simulink model "youhua_1226"  (R2017b)
settings: Solver=ode1  StartTime=0.0  StopTime=Inf  FixedStep=0.0002  RelTol=1e-3
PreLoadFcn:
  | initFun_4P.m
PostLoadFcn:
  | , if any(exist('dsrtsu_mdlpostloadfcn', 'file') == [2, 3, 6]), try dsrtsu_mdlpostloadfcn('Execute', bdroot); catch fprintf('Error in PostLoadFcn (dsrtsu_mdlpostloadfcn) for model "%s":\n %s\n', bdroot, lasterr); end, end,
InitFcn:
  | initFun_4P
undefined symbols (not defined in the file): CMAES_B_initial, CMAES_C_initial, CMAES_chiN_initial, CMAES_counteval_initial, CMAES_D_initial, CMAES_eigeneval_initial, CMAES_invsqrtC_initial, CMAES_pc_initial, CMAES_ps_initial, CMAES_sigma_initial, CMAES_xmean_initial
libraries: rti1202lib_adc_class1 x20, simulink x8, dsparch4 x6, rti1202serlib x4, rti1202lib_dio_class1 x4, dsextras x3, rtiemclib x2, rti1202lib_dac_class1 x1, rtitasklib x1
(part 5 of 6)

== matlab function youhua_1226/CONTROL/Control and Display/State Transition ==
  data: state_output output; stride_T output; buttons input; digital_inputs input; state_input input; analog_inputs input; user_inputs input; state_variables input; current_time input; ABL_user_inputs input; max_ankle_pos input; current_state_time output
function [state_output, stride_T, current_state_time] = fcn(buttons, digital_inputs, state_input,...
    analog_inputs, user_inputs, state_variables, current_time, ...
    ABL_user_inputs, max_ankle_pos)



%State definitions
idle_state	=	0;
calibration_state	=   1;
stance_state   =   2;
swing_state     =   3;
step_state  =   4;
slack_state = 5;
pos_track_state = 6;
%#eml

tracksize = 5;




foot_switch     =   digital_inputs(1);


bt_set_zero     =   buttons(1);
bt_walk         =   buttons(2);
bt_stop         =   buttons(3);
bt_step         =   buttons(4);
bt_slack        =   buttons(5);
bt_pos_test     =   buttons(6);

% measured_force = analog_inputs(4);
measured_force = state_variables(7);
ankle_pos = state_variables(3);
measured_torque = state_variables(6);

slack_force = user_inputs(5);
slack_length = user_inputs(22);
planter_low_limit = user_inputs(77);
walk_control_mode = user_inputs(21);

%当前状态持续时间
current_state_time = state_variables(21)-state_variables(23);

current_state = state_input(1);
stop_pos_prev = state_input(2);
slack_pos_prev = state_input(3);
stance_end_pos_prev = state_input(4);
stance_period_prev = state_input(5);
flag_dorsi_plantar_prev = state_input(6);
temp_ankle_pos1_prev = state_input(7);
temp_ankle_pos2_prev = state_input(8);
temp_ankle_pos3_prev = state_input(9);
temp_ankle_pos4_prev = state_input(10);
temp_ankle_pos5_prev = state_input(11);
stance_index_prev = state_input(12);
stride_time_prev = state_input(13);
step_start_time_prev = state_input(14);
dorsi_end_pos_prev = state_input(15);
ABL_ankle_index_prev = state_input(16);




state_output = state_input;
stop_pos = stop_pos_prev;
slack_pos = slack_pos_prev;
stance_end_pos = stance_end_pos_prev;
stance_period = stance_period_prev;
flag_dorsi_plantar = flag_dorsi_plantar_prev;
temp_ankle_pos1 = temp_ankle_pos2_prev;
temp_ankle_pos2 = temp_ankle_pos3_prev;
temp_ankle_pos3 = temp_ankle_pos4_prev;
temp_ankle_pos4 = temp_ankle_pos5_prev;
temp_ankle_pos5 = state_variables(3);
stance_index = stance_index_prev;
stride_time = stride_time_prev;
%---------------------
stride_T = stride_time;
%---------------------------
ABL_ankle_index = ABL_ankle_index_prev;

if(stride_time <0.7)
    stride_time = 0.7;
elseif(stride_time>1.5)
    stride_time =1.5;
end
step_start_time = step_start_time_prev;
dorsi_end_pos = dorsi_end_pos_prev;

ABL_ankle_min = ABL_user_inputs(1);
ABL_ankle_res = ABL_user_inputs(2);
ABL_or_TBL = ABL_user_inputs(3);


% ABL_ankle_index = stance_index_prev;
ABL_ankle_index = floor((ankle_pos-ABL_ankle_min)/ABL_ankle_res)+1;


switch current_state
    case idle_state
        if bt_set_zero  ==  1
            next_state = calibration_state;
        elseif bt_slack  == 1
            next_state = slack_state;
            slack_pos = state_variables(4);
        elseif bt_walk	==  1
            next_state = swing_state;
        elseif bt_step  ==  1
            next_state = step_state;
        elseif bt_pos_test ==1
            next_state = pos_track_state;
        else
            next_state = idle_state;
            %             stop_pos = state_variables(4);
        end
    case calibration_state
        if bt_stop == 1
            next_state = idle_state;
            stop_pos = state_variables(4);
        elseif measured_torque < slack_force % less than 2 lbs
            next_state = calibration_state;
        else
            next_state = idle_state;
            stop_pos = state_variables(4);
        end
    case stance_state
        %---------------

        %---------------
        if bt_stop	==	1
            next_state = idle_state;
            stop_pos = state_variables(4);
            flag_dorsi_plantar = 0;
        elseif bt_slack  == 1
            next_state = slack_state;
            slack_pos = state_variables(4);
            flag_dorsi_plantar = 0;
            %         elseif (current_state_time >=0.6*stride_time && temp_ankle_pos5<temp_ankle_pos4 && temp_ankle_pos5<temp_ankle_pos4 && measured_force<planter_low_limit)
%         elseif (current_state_time >=0.65*stride_time ||
%         ankle_pos>max_ankle_pos) $$$$$$$$$$
            elseif (current_state_time >=0.65*stride_time)
            next_state = swing_state;
            stance_end_pos = state_variables(4);
            stance_period = current_state_time;
            flag_dorsi_plantar = 0;
        elseif current_state_time<0.30*stride_time
            next_state = stance_state;
            stance_index = stance_index +1;
            flag_dorsi_plantar = 0;
        else
            stance_index = stance_index+1;
            next_state = stance_state;
            if flag_dorsi_plantar == 0
                if(temp_ankle_pos4>temp_ankle_pos3 && temp_ankle_pos5>temp_ankle_pos4)
                    flag_dorsi_plantar = 1;
                    dorsi_end_pos = state_variables(3);
                end
            end
        end
    case swing_state
        %---------

        %---------------
        
        if bt_stop == 1
            next_state = idle_state;
            stop_pos = state_variables(4);
        elseif bt_slack  == 1
            next_state = slack_state;
            slack_pos = state_variables(4);
        elseif foot_switch ==   1
            if current_state_time>0.15*stride_time
%                 if current_state_time>0.15

                next_state = stance_state;
                stance_index = 1;
                stride_time = (current_time - step_start_time+stride_time+stride_time_prev)/3;
                step_start_time = current_time;
            else
                next_state = swing_state;
            end
        else
            next_state = swing_state;
        end
    case step_state
        if bt_stop == 1
            next_state = idle_state;
            stop_pos = state_variables(4);
        elseif bt_slack  == 1
            next_state = slack_state;
            slack_pos = state_variables(4);
        else
            next_state = step_state;
        end
    case slack_state
        if bt_stop == 1
            next_state = idle_state;
            stop_pos = state_variables(4);
        elseif (abs(state_variables(4)-slack_pos-slack_length)<1)
            next_state = idle_state;
            stop_pos = state_variables(4);
        else
            next_state = slack_state;
        end
    case pos_track_state
        if bt_stop == 1
            next_state = idle_state;
            stop_pos = state_variables(4);
        elseif bt_slack  == 1
            next_state = slack_state;
            slack_pos = state_variables(4);
        else
            next_state = pos_track_state;
        end
    otherwise
        next_state  = current_state;
end

state_output(1) = next_state;
state_output(2) = stop_pos;
state_output(3) = slack_pos;
state_output(4) = stance_end_pos;
state_output(5) = stance_period;
state_output(6) = flag_dorsi_plantar;
state_output(7) = temp_ankle_pos1;
state_output(8) = temp_ankle_pos2;
state_output(9) = temp_ankle_pos3;
state_output(10) = temp_ankle_pos4;
state_output(11) = temp_ankle_pos5;

%     case 0
%         if flag_dorsi_planter==0
%         state_output(12) = ABL_ankle_index;
%         else
%             state_output(12) = ABL_ankle_index + 300;
%         end;
%     case 1
%     state_output(12) = stance_index;
%     otherwise
state_output(12) = stance_index;
state_output(13) = stride_time;
state_output(14) = step_start_time;
state_output(15) = dorsi_end_pos;
if flag_dorsi_plantar==0
    state_output(16) = ABL_ankle_index;
else
    state_output(16) = ABL_ankle_index + 300;
end
return

== matlab function youhua_1226/CONTROL/Control and Display/OutputBlock/Display and Recording ==
  data: current_state input; state output; state_variables input; motor_velocity input; desired_velocity output; zero_ankle_pos output; zero_motor_pos output; ankle_pos output; motor_pos output; desired_torque output; measured_torque output; load_force output; load_angle output; load_pivot_distance output; delta_motor_pos output; slack_motor_pos output; torque_error output; Kp output; ankle_vel output; motor_vel output; motor_acc output; Kd output; Ki output; controller_type output; Kc output; current_time output; state_start_time output; curve_id output; Kpp output; accumulated_torque_error output; desired_motor_pos output; walk_control_mode output; prev_step_accumulated_error output; curr_step_accumulated_error output; learning_control_input output; learning_control_input2 output; Kp2 output; Kl output; Kl2 output; flag_d_p output; gamma output; Lce output; Lmtu output; FL output; Fpe output; ACT output; STIM output; Fmtu output; Lcedot output; learned_value output; learned_avg output; accumulated_pos_error output; gamma1 output; gamma2 output; gamma3 output; gamma4 output
function [state, desired_velocity, zero_ankle_pos,  zero_motor_pos,...
    ankle_pos,motor_pos,desired_torque,measured_torque,load_force,...
    load_angle, load_pivot_distance,delta_motor_pos,slack_motor_pos,...
    torque_error, Kp, ankle_vel, motor_vel, motor_acc, Kd, Ki,...
    controller_type, Kc, current_time, state_start_time, curve_id, Kpp,...
    accumulated_torque_error, desired_motor_pos, walk_control_mode, ...
    prev_step_accumulated_error, curr_step_accumulated_error,...
    learning_control_input, learning_control_input2, Kp2, Kl,Kl2,...
    flag_d_p,gamma, Lce, Lmtu, FL, Fpe, ACT, STIM, Fmtu, Lcedot,...
    learned_value, learned_avg, accumulated_pos_error,...
    gamma1, gamma2, gamma3, gamma4]...
= fcn(current_state,state_variables, motor_velocity)

zero_ankle_pos  =  state_variables(1);
zero_motor_pos  = state_variables(2);
ankle_pos  = state_variables(3);
motor_pos  = state_variables(4);
desired_torque  = state_variables(5);
measured_torque  = state_variables(6);
load_force  = state_variables(7);
load_angle  = state_variables(8);
load_pivot_distance  = state_variables(9);
delta_motor_pos  = state_variables(10);
slack_motor_pos  = state_variables(11);
torque_error  = state_variables(12);
Kp = state_variables(13);
ankle_vel = state_variables(14);
motor_vel = state_variables(15);
motor_acc = state_variables(16);
Kd = state_variables(17);
Ki = state_variables(18);
controller_type = state_variables(19);
Kc = state_variables(20);
current_time = state_variables(21);
state_start_time = state_variables(23);
curve_id = state_variables(24);
Kpp = state_variables(25);
accumulated_torque_error= state_variables(26);
desired_motor_pos = state_variables(27);
walk_control_mode = state_variables(28);
prev_step_accumulated_error = state_variables(29);
curr_step_accumulated_error = state_variables(30);
learning_control_input= state_variables(31);
learning_control_input2 = state_variables(32);
Kp2 = state_variables(33);
Kl = state_variables(34);
Kl2 = state_variables(35);
flag_d_p = state_variables(36);
gamma = state_variables(37);
Lce = state_variables(38);
Lmtu = state_variables(39);
FL = state_variables(40);
Fpe = state_variables(41);
ACT = state_variables(42);
STIM = state_variables(43);
Fmtu = state_variables(44);
Lcedot = state_variables(45);
learned_value = state_variables(46);
learned_avg = state_variables(47);
accumulated_pos_error = state_variables(48);
gamma1 = state_variables(49);
gamma2 = state_variables(50);
gamma3 = state_variables(51);
gamma4 = state_variables(52);
state = current_state(1);
desired_velocity = motor_velocity;
return

== matlab function youhua_1226/CONTROL/Control and Display/time derivatives /MATLAB Function2 ==
  data: u input; desired_torque output; measured_torque output; desired_motor_pos output
function [desired_torque, measured_torque, desired_motor_pos] = fcn(u)
%#codegen

desired_torque = u(1);
measured_torque = u(2);
desired_motor_pos = u(3);

== matlab function youhua_1226/Serial Decoding System/Serial Data Processing ==
  data: serial_buffer_prev input; serial_buffer_next output; clk input; serial_data input; vdata_prev input; idx_prev input; buff_data_prev input; meta_E_prev input; t_prev input; vdata output; idx output; buff_data output; meta_E output; t output; trig output
function [serial_buffer_next, vdata, idx, buff_data, meta_E, t, trig]   = fcn(serial_buffer_prev, clk, serial_data, vdata_prev,...
    idx_prev, buff_data_prev, meta_E_prev, t_prev)
vdata = vdata_prev;
vo2_prev = vdata_prev(1);
vco2_prev = vdata_prev(2);
vo2 = vo2_prev;
vco2 = vco2_prev;
idx = idx_prev;
idx_o2_prev=idx_prev(1);
idx_co2_prev = idx_prev(2);

idx_o2 = idx_o2_prev;
idx_co2 = idx_co2_prev;

buff_data = buff_data_prev;
buff_vo2_prev = buff_data_prev(1,:);
buff_vco2_prev = buff_data_prev(2,:);
buff_vo2 = buff_vo2_prev;
buff_vco2 = buff_vco2_prev;

meta_E = meta_E_prev;
t = t_prev;

trig = 0;

serial_buffer_next = zeros(2,100);
serial_buffer_next = serial_buffer_prev;
idx_o2 = idx_o2+1;

serial_char = char(serial_data);
if serial_char == '#'
    idx_o2 = 1;
    temp_serial = zeros(2,100);
    temp_serial(1, idx_o2)= serial_char;
    serial_buffer_next = temp_serial;
    
    
    
    
    buff_vo2 = [0 0 0 0 0];
    % elseif serial_char == '~'
    %     %idx_o2 = -1;
    %     idx_co2 = 0;
    %     buff_vco2 = [0 0 0 0 0];
elseif serial_char == '!'
    temp_str = serial_buffer_prev(1, 1:idx_o2);
    iddx = find(temp_str=='~');
    str1 = temp_str(2:iddx(1)-1);
    str2 = temp_str(iddx(1)+1:idx_o2-1);
%     str3 = temp_str(iddx(2)+1:iddx(3)-1);
%     str4 = temp_str(iddx(3)+1:iddx(4)-1);
%     str5 = temp_str(iddx(4)+1:iddx(5)-1);
%     str6 = temp_str(iddx(5)+1:idx_o2-1);
    
    num1 = s2n(length(str1), str1);
    num2 = s2n(length(str2), str2);
%     num3 = s2n(length(str3), str3);
%     num4 = s2n(length(str4), str4);
%     num5 = s2n(length(str5), str5);
%     num6 = s2n(length(str6), str6);
    
%     if (num1==num3 || num1 == num5)
%         
%         vo2 = num1;
%         
%     elseif num3 == num5
%         vo2 = num3;
%     else
%         vo2 = -10000;
%         
%     end;
%     if (num2==num4 || num2 == num6)
%         
%         vco2 = num2;
%         
%     elseif num4 == num6
%         vco2 = num4;
%     else
%         vco2 = -20000;
%         
%     end;
    
    vo2 = num1;
    vco2 = num2;
    
    
    if vo2>0 && vco2>0
        meta_E = (16.477*vo2+4.484*vco2)/60;
        t = clk;
        trig = 1;
        
        idx_o2 = -1;
        idx_co2 = -1;
    end;
    % elseif idx_o2>=0 && idx_co2 <0
    %     idx_o2 = idx_o2+1;
    %     buff_vo2(idx_o2)=serial_char;
    % elseif idx_o2>=0 && idx_co2>=0
    %     idx_co2 = idx_co2+1;
    %     buff_vco2(idx_co2) = serial_char;
else
    temp_serial = zeros(2,100);
    temp_serial(1, 1:idx_o2) = serial_buffer_prev(1, 1:idx_o2);
    temp_serial(1, idx_o2)= serial_char;
    serial_buffer_next = temp_serial;
end;


vdata =[vo2;vco2];
idx = [idx_o2; idx_co2];
buff_data = [buff_vo2; buff_vco2];

return;


% function num  = s2n2(idx, char_arr)
% i = idx;
% num = 0;
% % char_arr = char_arr(end:1:1);
% for k=1:1:i
%     num = num + (double(char_arr(k))-48)*10^(i-k);
% end;

function num  = s2n(idx, char_arr)
num = 0;

arabic_arr_idx = find(char_arr~='@');

arabic_arr = char_arr(arabic_arr_idx);
i = length(arabic_arr);
% char_arr = char_arr(end:1:1);
for k=1:1:i
    if (arabic_arr(k)<45 || arabic_arr(k)>57 || arabic_arr(k)== 46 || arabic_arr(k)==47)
        num = -30000;
        break;
    else
        if arabic_arr(1)==45
            if k>1
                num = num -(double(arabic_arr(k))-48)*10^(i-k-1);
            end;
        else
            num = num + (double(arabic_arr(k))-48)*10^(i-k);
        end;
    end
end;

return;

== matlab function youhua_1226/Serial Decoding System/OODataGroupin ==
  data: metA input; optdata output; paramNo input; param input
function optdata = fcn(metA, paramNo, param)

optdata = zeros(6, 1);
optdata(1,1) = metA;
optdata(2,1) = paramNo;
optdata(3:end,1) = param;

== matlab function youhua_1226/Serial Decoding System/Metabolics Processing/Data Saving ==
  data: timeconstant input; met_array_out output; fakeMode input; fakeMetA input; newDatatrig input; dataPointDefMode input; start_opt input; stop_opt input; current_time input; data_pt_dur input; max_idx input; m_data input; met_array_in input; i_prev input; met_avg_prev input; fitted_met_avg_prev input; data_saving_status_prev input; period_start_time_prev input; i output; met_avg output; fitted_met_avg output; trig output; data_saving_status output; period_start_time output
function [ met_array_out, i, met_avg,fitted_met_avg, trig, data_saving_status,period_start_time]       = m_data_save(timeconstant, fakeMode, fakeMetA,newDatatrig, dataPointDefMode, start_opt, stop_opt, current_time, data_pt_dur,max_idx,...
    m_data, met_array_in,i_prev, met_avg_prev, fitted_met_avg_prev,data_saving_status_prev, period_start_time_prev)


i = i_prev;

met_avg = met_avg_prev;
fitted_met_avg = fitted_met_avg_prev;

trig = 0;
data_saving_status = data_saving_status_prev;
period_start_time = period_start_time_prev;
% isPaused = isPaused_prev;

if start_opt ==1;
    data_saving_status = 1;
    period_start_time = current_time;
    met_array_out = zeros(size(met_array_in));
    i = 0;
end;
if stop_opt  == 1
    data_saving_status =0;
    met_array_out = zeros(size(met_array_in));
    i = 0;
end;

% if pause_bn ==1;
%     isPaused = 1;
%     i = 0;
%     met_array_out = zeros(size(met_array_in));
% end;
% if unpause_bn  == 1
%     isPaused =0;
%     period_start_time = current_time;
% end;


time_this_dur = current_time - period_start_time;
% temp_data = zeros(2, 200);
if newDatatrig ==1
    
    if (data_saving_status==1)
        
        i = i+1;
        temp_data = met_array_in;
        temp_data(1, i) = m_data(1);
        temp_data(2, i) = time_this_dur;
        met_array_out = temp_data;
        
        
        switch dataPointDefMode
            case 0 % based on counts
                if i == max_idx
                    
                    met_avg = mean(met_array_out(1,1:i));
                    trig = 1;
                    if i>2
                        fitted_met_avg = sum(metabolicsMapping(met_array_out(2,1:i), ones(1,i), met_array_out(1,1:i), timeconstant,4));
                        if fitted_met_avg <=0
                            fitted_met_avg = met_avg;
                        end;
                    else
                        fitted_met_avg = met_avg;
                    end
                    % for debugging, manual input of met data
                    if fakeMode == 1
                        fitted_met_avg = fakeMetA;
                    end;
                    i = 0;
                    met_array_out = zeros(size(met_array_in));
                    period_start_time = current_time;
                end;
                
            case 1 % based on time
                
                if time_this_dur>=data_pt_dur
                    trig = 1;
                    met_avg = mean(met_array_out(1, 1:i));
                    if i>2
                        fitted_met_avg = sum(metabolicsMapping(met_array_out(2,1:i), ones(1,i), met_array_out(1,1:i), timeconstant, 4));
                        if fitted_met_avg <=0
                            fitted_met_avg = met_avg;
                        end;
                    else
                        fitted_met_avg = met_avg;
                        
                    end;
                    if fakeMode == 1
                        fitted_met_avg = fakeMetA;
                    end;
                    
                    i = 0;
                    met_array_out = zeros(size(met_array_in));
                    period_start_time = current_time;
                end
        end
        
    else
        
        met_array_out = met_array_in;
        
    end;
else
    met_array_out = met_array_in;
    
end;



return


function polyOut = metabolicsMapping(t,p,y_m,tau,n_deg)
if isrow(y_m)
    y_meas = y_m';
elseif iscolumn(y_m)
    y_meas = y_m;
else
    error('Measurements are not a single column vector')
    
end;

n_samp = length(t);
A = zeros(n_samp, n_deg+2);
A(1,:) = [1, zeros(1, n_deg+1)];
for i = 2:length(t)
    for j = 1:n_deg+2
        dt = t(i)-t(i-1);
        if j == 1
            A(i ,j) = A(i-1,j)*(1-dt/tau);
        else
            A(i ,j) = A(i-1,j)*(1-dt/tau) + (dt/tau)*p(i)^(j-2);
        end;
    end
end;
x_star = pinv(A)*y_meas;
y_bar = A*x_star;
mean_squared_error = ((y_bar-y_meas)'*(y_bar-y_meas))/n_samp;
polyOut = fliplr(x_star(2:end)');
return

== matlab function youhua_1226/CONTROL/Control and Display/changemonitor ==
  data: datain input; ischanged output; prev_data input; dataout output
function [ischanged, dataout]= fcn(datain, prev_data)

if ~isequal(datain, prev_data)
    ischanged = 1;
else
    ischanged = 0;
end

dataout = datain;

== matlab function youhua_1226/Serial Decoding System/Metabolics Processing/OO/optimization ==
  data: oo_dtau_offset input; OOParamNo output; maxTorque input; optTrig input; optData input; metA input; param input; noParam input; optAlgo input; OOReset input; CMAES_xmean_initials input; CMAES_sigma_initial input; CMAES_D_initials input; CMAES_B_initials input; idx_prev input; initCheck_prev input; noDataPoints_prev input; ameba_state_prev input; surrogate_state_prev input; cmaes_state_prev input; CMAES_pc_prev input; CMAES_ps_prev input; CMAES_B_prev input; CMAES_D_prev input; CMAES_C_prev input; CMAES_invsqrtC_prev input; CMAES_eigeneval_prev input; CMAES_chiN_prev input; CMAES_sigma_prev input; CMAES_counteval_prev input; CMAES_xmean_prev input; optData_next output; param_next output; idx output; initCheck output; noDataPoints output; ameba_state output; surrogate_state output; cmaes_state output; CMAES_pc output; CMAES_ps output; CMAES_B output; CMAES_D output; CMAES_C output; CMAES_invsqrtC output; CMAES_eigeneval output; CMAES_chiN output; CMAES_sigma output; CMAES_counteval output; CMAES_xmean output; initDataSize output; current_param output; CMAES_weights output; X2 output
function [OOParamNo, optData_next, param_next, idx, initCheck, noDataPoints,...
    ameba_state, surrogate_state, cmaes_state,...
    CMAES_pc, CMAES_ps, CMAES_B, CMAES_D, CMAES_C, CMAES_invsqrtC,...
    CMAES_eigeneval, CMAES_chiN, CMAES_sigma, CMAES_counteval,...
    CMAES_xmean,...
    initDataSize, current_param, CMAES_weights, X2]= optFun(oo_dtau_offset,maxTorque,optTrig,optData,metA,...
    param, noParam, optAlgo,  OOReset,...
    CMAES_xmean_initials, CMAES_sigma_initial, CMAES_D_initials,...
    CMAES_B_initials,...
    idx_prev, initCheck_prev,noDataPoints_prev,...
    ameba_state_prev, surrogate_state_prev, cmaes_state_prev,...
    CMAES_pc_prev, CMAES_ps_prev, CMAES_B_prev, CMAES_D_prev,...
    CMAES_C_prev, CMAES_invsqrtC_prev,...
    CMAES_eigeneval_prev, CMAES_chiN_prev, CMAES_sigma_prev,...
    CMAES_counteval_prev,CMAES_xmean_prev)
  


param_next = param;
current_param = param;
idx = idx_prev;
optData_next = optData;
initCheck = initCheck_prev;
noDataPoints = noDataPoints_prev;
ameba_state = ameba_state_prev;
surrogate_state = surrogate_state_prev;
cmaes_state = cmaes_state_prev;




CMAES_pc = CMAES_pc_prev;
CMAES_ps = CMAES_ps_prev;
CMAES_B = CMAES_B_prev;
CMAES_D = CMAES_D_prev;
CMAES_C = CMAES_C_prev;
CMAES_invsqrtC = CMAES_invsqrtC_prev;
CMAES_eigeneval = CMAES_eigeneval_prev;
CMAES_chiN = CMAES_chiN_prev;
CMAES_sigma = CMAES_sigma_prev;
CMAES_counteval = CMAES_counteval_prev;
CMAES_xmean= CMAES_xmean_prev;
CMAES_weights = zeros(4, 1);
assert(noParam<5);
OOParamNo = noParam;

X2 = zeros(8, 4);

%%ameba parameters
alpha = 1;
gamma = 2;
rho = 0.5;
sigma = 0.5;

switch optAlgo
    case 1 % ameba
        initDataSize = noParam+1;
        genSize = 1;
    case 2 & 3 % surrogate based, 2: fifo; 3: all available data
        initDataSize = noParam*2+noParam*(noParam-1)+1;
        genSize = 1;
    case 4
        initDataSize = 4+floor(3*log(noParam));
        genSize = initDataSize;
        
    otherwise
        initDataSize = noParam+1;
        genSize =1;
end;


if OOReset == 1
    InitialParams = zeros(8, 5);
    %for step frequency
    
    
    initCheck = 0;
    idx = 0;
    noDataPoints = 0; % # of
    
    
    ameba_state = 0;
    surrogate_state = 0;
    cmaes_state = 0;
    
    
    
    CMAES_pc = zeros(4,1);
    CMAES_ps = zeros(4,1);
    CMAES_B = eye(4,4);
    CMAES_D = ones(4,1);
    CMAES_C = CMAES_B * diag(CMAES_D.^2) * CMAES_B';
    CMAES_invsqrtC = CMAES_B * diag(CMAES_D.^-1) * CMAES_B';
    CMAES_eigeneval = 0;
    
    
    CMAES_counteval = 0;
    %     CMAES_xmean= zeros(15,1);
    
    CMAES_chiN = noParam^0.5*(1-1/(4*noParam)+1/(21*noParam^2));
    
    %     [CMAES_sigma, CMAES_xmean]=reset_param(noParam);
    if isrow(CMAES_xmean_initials)
        CMAES_xmean = CMAES_xmean_initials';
    else
        CMAES_xmean = CMAES_xmean_initials;
    end;
    
    CMAES_sigma = CMAES_sigma_initial;
    CMAES_D = CMAES_D_initials;
     CMAES_B = [CMAES_B_initials(1:4)';CMAES_B_initials(5:8)';CMAES_B_initials(9:12)';CMAES_B_initials(13:16)'];
     % CMAES_invsqrtC=CMAES_invsqrtC_initial;%%%%%%%%%%%%%%%%%%%%%%%%%%%
    %         CMAES_xmean(1,1)=1.1;
    %     CMAES_sigma = 0.1;
    
    
    B = CMAES_B(1:noParam, 1:noParam);
    D = CMAES_D(1:noParam, 1);
    
    sigma  = CMAES_sigma;
    xmean = CMAES_xmean(1:noParam,1);
    
    
    assert(noParam<5)
    assert(initDataSize < 8);
    initx = zeros(noParam, initDataSize);
    
    switch optAlgo
        case 1
            
            for k=1:initDataSize,
                initx(:,k) = xmean + sigma * B * (D .* randn(noParam,1)); % m + sig * Normal(0,C)
                %                         x3(:,k) = xmean + sigma*C*randn(noParam,1); % m + sig * Normal(0,C)
                if noParam==4
                initx(:,k) = applyConstraints(initx(:,k), maxTorque, oo_dtau_offset);
                end;                
            end
            
        case 4     
            
            for k=1:initDataSize,
                initx(:,k) = xmean + sigma * B * (D .* randn(noParam,1)); % m + sig * Normal(0,C)
                %                         x3(:,k) = xmean + sigma*C*randn(noParam,1); % m + sig * Normal(0,C)
                if noParam==4
                initx(:,k) = applyConstraints(initx(:,k), maxTorque,oo_dtau_offset);
                end;
            end
            
            
        otherwise
    end;
    
    % constraint parameters
    
    initx(find(initx<0))=0;
    
    % sort parameters according to parameter 1, the peak desired torque,
    
    [~, iii] = sort(initx(1, :));
    initx = initx(:, iii);
    

    InitialParams(1:initDataSize,2:noParam+1) = initx';
    
  
    optData_next = InitialParams;
    param_next = zeros(size(param_next));
    param_next(1:noParam,1) = (optData_next(noDataPoints+1, 2:noParam+1))';
    
else
    
    %% update onlly when triggered
    if optTrig ==1
        idx = idx +1; % increase data point count
        
        if initCheck == 0 % initial data collection
            if idx<=initDataSize
                temp = optData;
                temp(idx, 2:noParam+1) = (param(1:noParam))';
                temp(idx, 1) = metA;
                optData_next = temp;
                %             noDataPoints = noDataPoints+1;
                param_next(1:noParam,1) = (optData(idx+1, 2:noParam+1))';
                %                 optData_next(end, 2:noParam+1) = param_next(1:noParam,1)';
                if idx == initDataSize
                    initCheck = 1;
                    ameba_state = 1;
                    surrogate_state = 1;
                    cmaes_state = 1;
                    idx = 0;
                end;
                
            end;
        end;
        
        
        if initCheck == 1
            
            switch optAlgo
                
                case 1 % ameba
                    
                    
                    noDataPoints = noParam+1; % # of points in memory
                    x = optData(1:noDataPoints,2:noParam+1); % all parameter values
                    y = optData(1:noDataPoints,1); % all cost function values
                    [y2, i2] = sort(y); % sort cost
                    x2 = x(i2, :); % parameter values in increasing order of cost
                    X2(1:noDataPoints, 1:noParam) = x2;
                    x0 = mean(x2(1:noDataPoints-1, :)); % centroid of all points exact the last one with highest y
                    xr = x0+alpha*(x0-x2(noDataPoints, :)); %reflected point
                    
                    switch ameba_state
                        
                        case 1 % first parameter point from optimization, the reflected point, new data already saved
                            
                            x(noDataPoints, :) = param(1:noParam,1)';
                            y(noDataPoints, 1) = metA;
                            
                            [y5, i5] = sort(y); % sort cost
                            x5 = x(i5, :); % parameter values in increasing order of cost
                            X2(1:noDataPoints, 1:noParam) = x5;
                            x05 = mean(x5(1:noDataPoints-1, :)); % centroid of all points exact the last one with highest y
                            xr5 = x05+alpha*(x05-x5(noDataPoints, :)); %reflected point
                            xr5(find(xr5<0))=0;
                            if noParam==4
                                temp_xr = applyConstraints(xr5', maxTorque, oo_dtau_offset);
                                xr5 = temp_xr';
                            end;
                            param_next(1:noParam,1) = xr5';
                            ameba_state = 2;
                        case 2 % compare new point with those in memory, noDataPoints count of data point in memory, and 1 new data point
                            if metA>=y2(1) && metA<y2(noDataPoints-1)
                                y2(noDataPoints,1) = metA;
                                x2(noDataPoints, :) = param(1:noParam,1)';
                                ameba_state = 2;
                                %                             tempx = (optData_next(1:noDataPoints,2:noParam+1))';
                                %                             tempy = (optData_next(1:noDataPoints,1))' ;
                                %                             tempx0 = zeros(size(tempx(:,1)));
                                [y3, i3] = sort(y2);
                                x3 = x2(i3, :);
                                
                                x02= mean(x3(1:noDataPoints-1, :));
                                
                                xr2 = x02+alpha*(x02-x3(noDataPoints, :));
                                xr2(find(xr2<0))=0;
                                if noParam==4
                                    temp_xr = applyConstraints(xr2', maxTorque, oo_dtau_offset);
                                    xr2 = temp_xr';
                                end;
                                param_next(1:noParam, 1) = xr2';
                                
                            elseif metA<y2(1)
                                xe = x0+gamma*(xr-x0);
                                xe(find(xe<0))=0;
                                if noParam==4
                                    temp_xr = applyConstraints(xe', maxTorque, oo_dtau_offset);
                                    xe = temp_xr';
                                end;
                                param_next(1:noParam, 1) = xe';
                                ameba_state = 3;
                                
                                % temp saving of reflected data point in memory
                                optData_next(noDataPoints+1, 2:noParam+1) = param(1:noParam,1)';
                                optData_next(noDataPoints+1, 1) = metA;
                            else % f(xr)>=f(x_n)
                                if metA>=y2(noDataPoints, 1)
                                    xc = x0+rho*(x2(noDataPoints,:)-x0);
                                else
                                    xc = x0+rho*(xr-x0);
                                end
                                xc(find(xc<0))=0;
                                if noParam==4
                                    temp_xr = applyConstraints(xc', maxTorque, oo_dtau_offset);
                                    xc = temp_xr';
                                end;
                                param_next(1:noParam,1) = xc';
                                ameba_state = 4;
                            end;
                            
                            optData_next(1:noDataPoints, 2:noParam+1) = x2;
                            optData_next(1:noDataPoints, 1) = y2;
                            %                             optData_next(end, 2:noParam+1) = param_next(1:noParam, 1)';
                            
                        case 3 % expanded point evaluated
                            if metA<optData(noDataPoints+1, 1)
                                y2(noDataPoints,1) = metA;
                                x2(noDataPoints, :) = param(1:noParam,1)'; %%% not working
                                
                            else
                                y2(noDataPoints,1) = optData(noDataPoints+1, 1);
                                x2(noDataPoints, :) = optData(noDataPoints+1, 2:noParam+1);
                                
                            end;
                            
                            optData_next(1:noDataPoints, 2:noParam+1) = x2;
                            optData_next(1:noDataPoints, 1) = y2;
                            
                            
                            [y3, i3] = sort(y2);
                            x3 = x2(i3, :);
                            
                            x02= mean(x3(1:noDataPoints-1, :));
                            
                            xr2 = x02+alpha*(x02-x3(noDataPoints,:));
                            xr2(find(xr2<0))=0;
                            if noParam==4
                                temp_xr = applyConstraints(xr2', maxTorque, oo_dtau_offset);
                                xr2 = temp_xr';
                            end;
                            param_next(1:noParam, 1) = xr2';
                            ameba_state = 2;
                            %                             optData_next(end, 2:noParam+1) = param_next(1:noParam, 1)';
                        case 4
                            if metA<y2(noDataPoints,1)
                                
                                y2(noDataPoints,1) = metA;
                                x2(noDataPoints, :) = param(1:noParam,1)';
                                optData_next(1:noDataPoints, 2:noParam+1) = x2;
                                optData_next(1:noDataPoints, 1) = y2;
                                
                                
                                [y3, i3] = sort(y2);
                                x3 = x2(i3,:);
                                
                                x02= mean(x3(1:noDataPoints-1, :));
                                
                                xr2 = x02+alpha*(x02-x3(noDataPoints, :));
                                xr2(find(xr2<0))=0;
                                if noParam==4
                                    temp_xr = applyConstraints(xr2', maxTorque, oo_dtau_offset);
                                    xr2 = temp_xr';
                                end;
                                param_next(1:noParam, 1) = xr2';
                                ameba_state = 2;
                            else
                                for i=2:1:(noParam+1)
                                    x2(i,:)= x2(1,:)+sigma*(x2(i,:)-x2(1,:));
                                    if noParam ==4
                                    temp_xr=applyConstraints(x2(i,:)', maxTorque, oo_dtau_offset);
                                    x2(i,:) = temp_xr';
                                    end;

                                end;
                                x2(find(x2<0))=0;

                                optData_next(1:noDataPoints,2:noParam+1) = x2;
                                optData_next(1:noDataPoints, 1) = y2;
                                
                                noDataPoints = 1;
                                initCheck = 0;
                                ameba_state = 0;
                                
                                surrogate_state = 0;
                                cmaes_state = 0;
                                idx = 1;
                                param_next(1:noParam,1) = x2(2, :)';
                            end;
                            %                             optData_next(end, 2:noParam+1) = param_next(1:noParam, 1)';
                        otherwise
                    end;
                case 2
                    %                 x3 = x2;
                    %                 y3 = y2;
                    %                 polyfit(x2(1,:), y2, 2);
                    
                case 3
                    %                 switch surrogate_state
                    %                     case 1
                    %                     case 2
                    %                     case 3
                    %                     otherwise
                    %                 end;
                case 4
                    
                    
                    
                    noDataPoints = initDataSize; % # of points in memory
                    x = optData(1:noDataPoints,2:noParam+1); % all parameter values
                    y = optData(1:noDataPoints,1); % all cost function values
                    x(noDataPoints, :) = param(1:noParam,1)';
                    y(noDataPoints, 1) = metA;
                    
                    [y2, i2] = sort(y); % sort cost
                    x2 = x(i2, :); % parameter values in increasing order of cost
                    X2(1:noDataPoints, 1:noParam) = x2;
                    x22 = x2'; %x in column
                    lambda = initDataSize;
                    assert(lambda<=8);
                    mu=lambda/2;
                    
                    
                    temp_w = zeros(4,1);
                    mu = floor(mu);
                    for j=1:1:mu
                        temp_w(j) = log(mu+1/2)-log(j);
                    end
                    
                    weights = temp_w(1:mu)/sum(temp_w(1:mu));
                    CMAES_weights(1:mu,1) = weights;
                    
                    mueff = sum(weights)^2/sum(weights.^2);
                    
                    cc = (4+mueff/noParam)/(noParam+4+2*mueff/noParam);
                    cs = (mueff+2) / (noParam+mueff+5);
                    c1 = 2 / ((noParam+1.3)^2+mueff);
                    cmu=min(1-c1, 2*(mueff-2+1/mueff)/((noParam+2)^2+mueff));
                    damps = 1 + 2*max(0, sqrt((mueff-1)/(noParam+1))-1)+cs;
                    
                    pc = CMAES_pc(1:noParam, 1);
                    ps = CMAES_ps(1:noParam, 1);
                    %                     B = zeros(noParam, noParam);
                    %                     D = zeros(noParam, 1);
                    %                     C = zeros(noParam, noParam);
                    B = CMAES_B(1:noParam, 1:noParam);
                    D = CMAES_D(1:noParam, 1);
                    C = CMAES_C(1:noParam, 1:noParam);
                    eigeneval = CMAES_eigeneval;
                    chiN =CMAES_chiN;
                    sigma  = CMAES_sigma;
                    counteval = CMAES_counteval;
                    xold = CMAES_xmean(1:noParam,1);
                    invsqrtC = CMAES_invsqrtC(1:noParam, 1:noParam);
                    
                    counteval = counteval+lambda;
%                     xold  = xmean;
                    %updates;
                    
                    xmean = zeros(noParam, 1);
                    for h=1:1:noParam
                        xmean(h, 1) = x22(h, 1:mu)*weights;
                    end;
                    
%                     xmean = x22(:, 1:mu)*weights;
                    
                    
                    
                    ps = (1-cs)*ps ...
                        + sqrt(cs*(2-cs)*mueff) * invsqrtC * (xmean-xold) / sigma;
                    hsig = norm(ps)/sqrt(1-(1-cs)^(2*counteval/lambda))/chiN < 1.4 + 2/(noParam+1);
                    pc = (1-cc)*pc ...
                        + hsig * sqrt(cc*(2-cc)*mueff) * (xmean-xold) / sigma;
                    
                    %                     assert(mu<20);
                    artmp = (1/sigma) * (x22(:,1:mu)-repmat(xold,1,mu));
                    C = (1-c1-cmu) * C ...                  % regard old matrix
                        + c1 * (pc*pc' ...                 % plus rank one update
                        + (1-hsig) * cc*(2-cc) * C) ... % minor correction if hsig==0
                        + cmu * artmp * diag(weights) * artmp'; % plus rank mu update
                    
                    % Adapt step size sigma
                    sigma = sigma * exp((cs/damps)*(norm(ps)/chiN - 1));
                    if counteval - eigeneval > lambda/(c1+cmu)/noParam/10  % to achieve O(N^2)
                        eigeneval = counteval;
                        C_tmp = triu(C) + triu(C,1)'; % enforce symmetry
                        [B,D_tmp] = eig(C_tmp);           % eigen decomposition, B==normalized eigenvectors
                        
                        D = sqrt(diag(D_tmp));        % D is a vector of standard deviations now
                        B = real(B);
                        D = real(D);
                        invsqrtC = B * diag(D.^-1) * B'; % to be fixed
                    end
                    
                    
                    CMAES_pc(1:noParam, 1) = pc;
                    CMAES_ps(1:noParam, 1) = ps;
                    CMAES_B(1:noParam, 1:noParam) = B; % to be fixed
                    CMAES_D(1:noParam, 1)=D(1:noParam, 1);% to be fixed
                    CMAES_C(1:noParam, 1:noParam)=C;
                    CMAES_eigeneval=eigeneval;
                    CMAES_chiN=chiN;
                    CMAES_sigma=sigma;
                    CMAES_counteval=counteval;
                    CMAES_xmean(1:noParam,1)=xmean;
                    CMAES_invsqrtC(1:noParam, 1:noParam) =invsqrtC;
                    
                    
                    initCheck = 0;
                    
                    
                    
                    x3 = zeros(noParam, lambda);
                    for k=1:lambda,
                        x3(:,k) = xmean + sigma * B * (D .* randn(noParam,1)); % m + sig * Normal(0,C)
                        if noParam == 4
                            temp_xr= applyConstraints(x3(:,k), maxTorque, oo_dtau_offset);
                            x3(:,k) = temp_xr;
                        end;
                        %                         x3(:,k) = xmean + sigma*C*randn(noParam,1); % m + sig * Normal(0,C)
                    end
                    %%
                    
                    x3(find(x3<0))=0;
                    

                    % sort parameters according to parameter 1, the peak desired torque,
                    
                    [~, iii] = sort(x3(1, :));
                    x3 = x3(:, iii);
                    %%
                    
                    optData_next(1:noDataPoints,2:noParam+1) = x3';
                    optData_next(1:noDataPoints,1) = zeros(noDataPoints,1);
                    
                    param_next(1:noParam) = x3(:,1);
                    
                    %                 switch cmaes_state
                    %                     case 1
                    %                     case 2
                    %                     case 3
                    %                     otherwise
                    %                 end;
                otherwise
            end;
        end;
        
    end;
end;
return;


function params = applyConstraints(original_params, maxTorque, oo_dtau_offset)
params = zeros(length(original_params), 1);

% assert params to be column vector;
if iscolumn(original_params)
    params = original_params;
else
    params = original_params';
end;


params(find(params<0))=0;
params(3,1) = max(10, params(3,1)); % rise time at least 10%
params(4,1) = max(10, params(4,1)); % drop time at least 5%
params(4,1) = min(40, params(4,1)); % drop time at most 20%
params(3,1) = min(40, params(3,1)); % drop time at most 20%

%% max peak desired torque 100Nm
params(1,1) = min(maxTorque-oo_dtau_offset, params(1,1));

peakTorque = params(1,1)+oo_dtau_offset;
if peakTorque < 0.75*maxTorque
    maxParam2 = 110;
else
    maxParam2 = 110-10*(peakTorque-0.75*maxTorque)/(0.25*maxTorque);
end;

params(2,1) = min(maxParam2, max(20,params(2,1)));

%% max peak 
% if params(2,1)/2>60
%     params(2,1)=120;
% end;
% if peak time + drop time go beyong 65%stride, shorten drop time; then
% lower limit 
if params(4,1)/2+params(2,1)/2>65
%     params(2,1)=2*(65-params(4,1)/2);
    params(4,1) = max(2*(65-params(2,1)/2),10);
end;
% if torque starts too early, reduce rise time
if params(2,1)/2-params(3,1)<5
    params(3,1) = max(params(2,1)/2-5, 10);
%     params(2,1)=2*(params(3,1)+5);
end;


return;

== matlab function youhua_1226/CONTROL/Control and Display/ooParmSampleHold/MATLAB Function ==
  data: u input; y output
function y = fcn(u)

y = u;
